simulink model "calibration_sensors"  (R2026a)
settings: Solver=VariableStepAuto  StopTime=inf
StopFcn:
  | coefficients = out.coefficients;
  | sensor_low = out.sensor_low;
  | sensor_high = out.sensor_high;
  | 
  | save('sensor_calibration.mat', ...
  |      'coefficients', ...
  |      'sensor_low', ...
  |      'sensor_high');
(part 3 of 3)

== matlab function calibration_sensors/MATLAB Function ==
  data: finished1 output; finished2 output; finished3 output; sh output; conflow1 input; confhigh1 input; conflow2 input; confhigh2 input; conflow3 input; confhigh3 input; aclow input; achigh input; adc1 input; c output; adc2 input; adc3 input; sl output
function [finished1, finished2, finished3, sh, c, sl] = fcn( ...
    conflow1, confhigh1, ...
    conflow2, confhigh2, ...
    conflow3, confhigh3, ...
    aclow, achigh, ...
    adc1, adc2, adc3)

persistent sensor_low sensor_high val_low val_high

if isempty(sensor_low)
    sensor_low  = zeros(3,1);
    sensor_high = zeros(3,1);

    val_low  = zeros(3,1);
    val_high = zeros(3,1);
end

% -------- Tank 1 --------
if conflow1 == 1
    sensor_low(1) = adc1;
    val_low(1) = 1;
end

if confhigh1 == 1
    sensor_high(1) = adc1;
    val_high(1) = 1;
end

% -------- Tank 2 --------
if conflow2 == 1
    sensor_low(2) = adc2;
    val_low(2) = 1;
end

if confhigh2 == 1
    sensor_high(2) = adc2;
    val_high(2) = 1;
end

% -------- Tank 3 --------
if conflow3 == 1
    sensor_low(3) = adc3;
    val_low(3) = 1;
end

if confhigh3 == 1
    sensor_high(3) = adc3;
    val_high(3) = 1;
end

% -------- Calculate calibration coefficients --------
c = zeros(3,1);

if val_low(1) == 1 && val_high(1) == 1 && sensor_high(1) ~= sensor_low(1)
    c(1) = (achigh - aclow) / (sensor_high(1) - sensor_low(1));
end

if val_low(2) == 1 && val_high(2) == 1 && sensor_high(2) ~= sensor_low(2)
    c(2) = (achigh - aclow) / (sensor_high(2) - sensor_low(2));
end

if val_low(3) == 1 && val_high(3) == 1 && sensor_high(3) ~= sensor_low(3)
    c(3) = (achigh - aclow) / (sensor_high(3) - sensor_low(3));
end

% -------- Outputs --------
sl = sensor_low;
sh = sensor_high;

finished = val_low & val_high;

finished1 = finished(1);
finished2 = finished(2);
finished3 = finished(3);
